simulink subsystem "myTHD_fixed"  (R2024a)
settings: Solver=VariableStepAuto  StartTime=0.0  StopTime=10.0  RelTol=1e-3
values from neighbouring files (symbols this model uses):
  BUFFER_LEN = 2048    [workspace.mat]
  MAIN_FREQ_INDEX = 9    [workspace.mat]
libraries: dspsigops x3, embmathops x1, dspswit3 x1, hdlsllib x1, simulink_extras x1
settings Model: Creator=Jan Rosa  LastModifiedBy=Jan Rosa

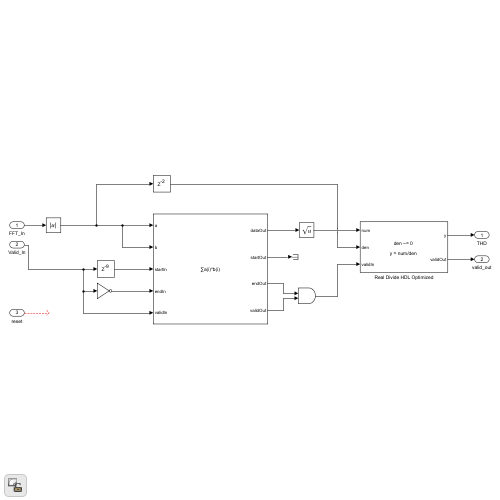
[thumbnail: Simulink's stored preview of the top-level diagram]
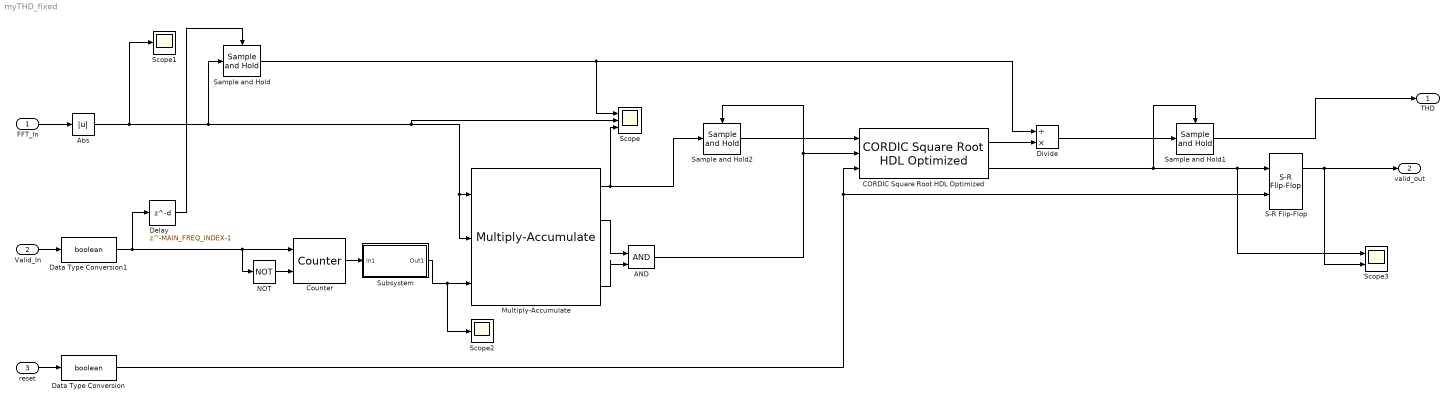
== system myTHD_fixed ==
  FFT_In : Inport
  Valid_In : Inport  Port=2
  reset : Inport  Port=3
  AND : Logic  IconShape=distinctive  AllPortsSameDT=off  OutDataTypeStr=boolean
  Abs : Abs  OutDataTypeStr=double  SaturateOnIntegerOverflow=off
  CORDIC Square Root HDL Optimized : embmathops/CORDIC Square Root HDL Optimized  autoMaximumShiftVal=on  maximumShiftValue=10  nIterPerReg=1
      settings: LibrarySourceBlock=embeddedMatrixLib/Math Operations/CORDIC Square Root HDL Optimized
  Counter : dspswit3/Counter  Direction=Up  CountEvent=Non-zero sample  CounterSize=User defined  MaxCount=BUFFER_LEN  InitialCount=0  Output=Count  HitValue=BUFFER_LEN/2-MAIN_FREQ_INDEX  ResetInput=on  SamplesPerFrame=1  Ts=1  CntDtype=double  HitDtype=Logical
  Data Type Conversion : DataTypeConversion  OutDataTypeStr=boolean  SaturateOnIntegerOverflow=off  RndMeth=Floor
  Data Type Conversion1 : DataTypeConversion  OutDataTypeStr=boolean  SaturateOnIntegerOverflow=off  RndMeth=Floor
  Delay : Delay  DelayLength=MAIN_FREQ_INDEX-1
  Divide : Product  Inputs=/*
  Multiply-Accumulate : hdlsllib/HDL Operations/Multiply-Accumulate  opMode=Streaming - using Number of Samples  initValueSetting=Dialog  initValue=0  initValueSetting2=Dialog  initValue2=0  initValueSetting3=Dialog  initValue3=0  num_samples=BUFFER_LEN/2-MAIN_FREQ_INDEX  RndMeth2=Floor  RndMeth3=Floor  datatype2=Inherit: Inherit via back propagation  datatype3=Inherit: Inherit via back propagation  validOut=on  endInandOut=on  startOut=on  countOut=on  dim=-1  DoSatur=off  parallel=off
  NOT : Logic  Operator=NOT  IconShape=distinctive  AllPortsSameDT=off  OutDataTypeStr=boolean
  S-R Flip-Flop : simulink_extras/Flip Flops/S-R Flip-Flop  initial_condition=0
  Sample and Hold : dspsigops/Sample and Hold  trig=Rising edge  initCond=0  latchinput=off
  Sample and Hold1 : dspsigops/Sample and Hold  trig=Rising edge  initCond=0  latchinput=off
  Sample and Hold2 : dspsigops/Sample and Hold  trig=Rising edge  initCond=0  latchinput=off
  Scope : Scope  NumInputPorts=3
  Scope1 : Scope
  Scope2 : Scope
  Scope3 : Scope  NumInputPorts=2
  Subsystem : Subsystem
  THD : Outport
  valid_out : Outport  Port=2
  wires:
  FFT_In/1 -> Abs/1
  Abs/1 -> Sample and Hold/1, Multiply-Accumulate/2, Multiply-Accumulate/1, Scope/2, Scope1/1
  Multiply-Accumulate/2 -> AND/1
  Multiply-Accumulate/1 -> Sample and Hold2/1, Scope/3
  Multiply-Accumulate/4 -> AND/2
  AND/1 -> CORDIC Square Root HDL Optimized/2, Sample and Hold2/Trigger
  Sample and Hold/1 -> Divide/1, Scope/1
  reset/1 -> Data Type Conversion/1
  CORDIC Square Root HDL Optimized/1 -> Divide/2
  Data Type Conversion1/1 -> Delay/1, Counter/1, NOT/1
  Divide/1 -> Sample and Hold1/1
  Sample and Hold1/1 -> THD/1
  CORDIC Square Root HDL Optimized/2 -> Sample and Hold1/Trigger, S-R Flip-Flop/1, Scope3/1
  Sample and Hold2/1 -> CORDIC Square Root HDL Optimized/1
  Valid_In/1 -> Data Type Conversion1/1
  Data Type Conversion/1 -> CORDIC Square Root HDL Optimized/3, S-R Flip-Flop/2
  Counter/1 -> Subsystem/1(In1)
  Subsystem/1(Out1) -> Scope2/1, Multiply-Accumulate/3
  NOT/1 -> Counter/2
  S-R Flip-Flop/1 -> valid_out/1, Scope3/2
  Delay/1 -> Sample and Hold/Trigger

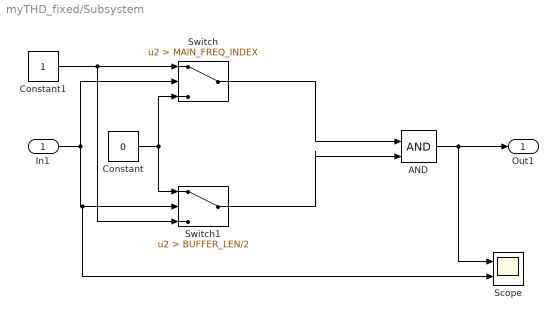
== system myTHD_fixed/Subsystem ==
  In1 : Inport
  AND : Logic  IconShape=distinctive  AllPortsSameDT=off  OutDataTypeStr=boolean
  Constant : Constant  Value=0
  Constant1 : Constant
  Scope : Scope  NumInputPorts=2
  Switch : Switch  Criteria=u2 > Threshold  Threshold=MAIN_FREQ_INDEX  SaturateOnIntegerOverflow=off  InputSameDT=off
  Switch1 : Switch  Criteria=u2 > Threshold  Threshold=BUFFER_LEN/2  SaturateOnIntegerOverflow=off  InputSameDT=off
  Out1 : Outport
  wires:
  Switch/1 -> AND/1
  Switch1/1 -> AND/2
  AND/1 -> Out1/1, Scope/1
  Constant1/1 -> Switch/1, Switch1/3
  Constant/1 -> Switch1/1, Switch/3
  In1/1 -> Switch/2, Switch1/2, Scope/2
